simulink model "drone_obs"  (R2022a)
settings: Solver=VariableStepAuto  StartTime=0.0  StopTime=20  RelTol=1e-3
undefined symbols (not defined in the file): a1, a2, a3
settings Model: Creator=dfcpstage6  LastModifiedBy=dfcpstage6
settings DebuggingCC: UnconnectedInputMsg=warning  UnconnectedOutputMsg=warning  UnconnectedLineMsg=warning
settings RTWCC: DLArmComputeVersion=19.05

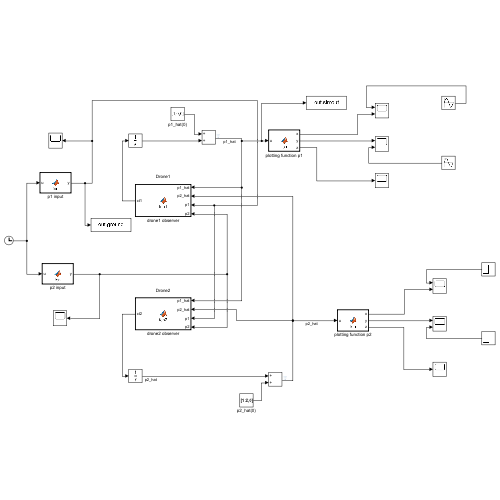
[thumbnail: Simulink's stored preview of the top-level diagram]
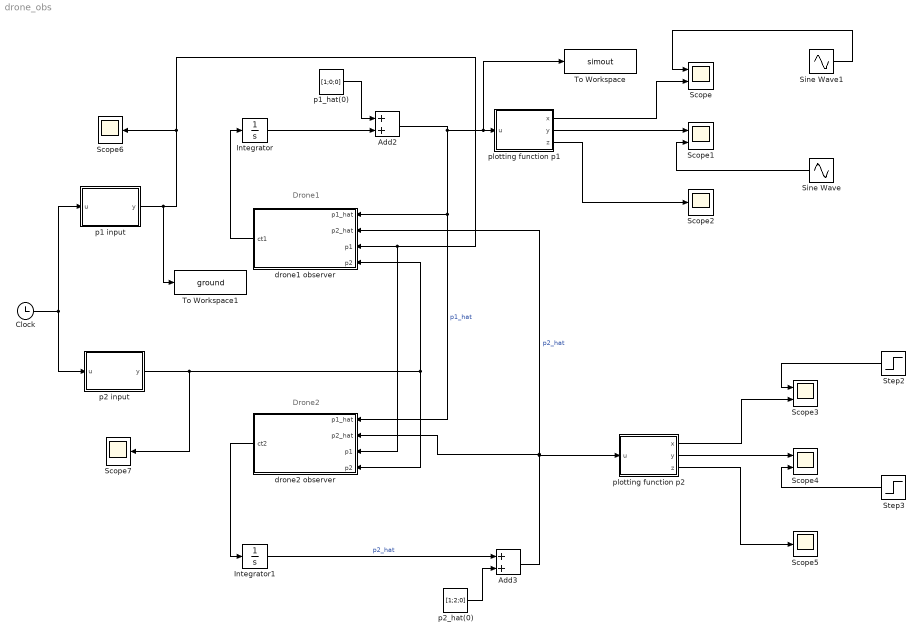
== system drone_obs ==
  note: Drone2
  note: Drone1
  Add2 : Sum
  Add3 : Sum
  Clock : Clock
  Integrator : Integrator
  Integrator1 : Integrator
  Scope{,1,3..4} (4 alike) : Scope  NumInputPorts=2
  Scope{2,5..7} (4 alike) : Scope
  Sine Wave : Sin  SampleTime=0
  Sine Wave1 : Sin  Phase=1.57  SampleTime=0
  Step2 : Step  Time=0.1  After=2  SampleTime=0
  Step3 : Step  Time=0.1  After=2  SampleTime=0
  To Workspace : ToWorkspace  VariableName=simout  SampleTime=-1
  To Workspace1 : ToWorkspace  VariableName=ground  SampleTime=-1
  drone1 observer : MATLAB Function  TreatAsAtomicUnit=on
  drone2 observer : MATLAB Function  TreatAsAtomicUnit=on
  p1 input : MATLAB Function  TreatAsAtomicUnit=on  SystemSampleTime=0.1
  p1_hat(0) : Constant  Value=[1;0;0]  VectorParams1D=off
  p2 input : MATLAB Function  TreatAsAtomicUnit=on  SystemSampleTime=0.1
  p2_hat(0) : Constant  Value=[1;2;0]  VectorParams1D=off
  plotting function p1 : MATLAB Function  TreatAsAtomicUnit=on
  plotting function p2 : MATLAB Function  TreatAsAtomicUnit=on
  wires:
  drone1 observer/1(ct1) -> Integrator/1
  drone2 observer/1(ct2) -> Integrator1/1
  Integrator/1 -> Add2/2
  Add2/1 -> drone2 observer/1(p1_hat), drone1 observer/1(p1_hat), To Workspace/1, plotting function p1/1(u)  "p1_hat"
  Integrator1/1 -> Add3/1  "p2_hat"
  p2_hat(0)/1 -> Add3/2
  p1_hat(0)/1 -> Add2/1
  plotting function p1/2(y) -> Scope1/1
  plotting function p1/3(z) -> Scope2/1
  plotting function p1/1(x) -> Scope/2
  p2 input/1(y) -> Scope7/1, drone1 observer/4(p2), drone2 observer/4(p2)
  p1 input/1(y) -> To Workspace1/1, drone2 observer/3(p1), drone1 observer/3(p1), Scope6/1
  plotting function p2/2(y) -> Scope4/1
  plotting function p2/3(z) -> Scope5/1
  Step2/1 -> Scope3/1
  Step3/1 -> Scope4/2
  plotting function p2/1(x) -> Scope3/2
  Add3/1 -> drone1 observer/2(p2_hat), drone2 observer/2(p2_hat), plotting function p2/1(u)  "p2_hat"
  Clock/1 -> p2 input/1(u), p1 input/1(u)
  Sine Wave1/1 -> Scope/1
  Sine Wave/1 -> Scope1/2

== matlab function drone_obs/drone2 observer ==
  data: p1_hat input; p2_hat input; ct2 output; a2 parameter; a3 parameter; p1 input; p2 input; a1 parameter
function ct2 = fcn2(p1_hat, p2_hat,a2, a3, p1, p2, a1)

% vel2 considering the second drone is just hovering in 2d space
    vel2 = [0;0;0];
%     vel2 = [2-p2(2); p2(1)-2 ;0];
    
%calculating the ranges manually
    d11 = norm(p1-a1);
    d13 = norm(p1-a3);
    d22 = norm(p2-a2);
    d23 = norm(p2-a3);
    q12 = norm(p1-p2);
    q21 = norm(p1-p2);
    
% our measured values
    y12 = d22^2 - d23^2 + norm(a3)^2 - norm(a2)^2;
    y22 = d23^2 + d13^2 - q21^2 - 2*norm(a3)^2;
    c23 = a3 - a2;
    
% controller gains
    k12 = c23;
    k22 = p1_hat - a3;
    
% correction terms
    ct2_1 = k12*(y12 - 2*(c23.')*p2_hat); 
    ct2_2 = k22*(y22 + 2*(a3.')*(p1_hat + p2_hat) - 2*(p1_hat.')*(p2_hat));
ct2 = vel2 + 1*ct2_1 + 1*ct2_2;

== matlab function drone_obs/drone1 observer ==
  data: p1_hat input; p2_hat input; ct1 output; p1 input; p2 input; a1 parameter; a2 parameter; a3 parameter
% function ct1 = fcn1(p1_hat, p2_hat ,a1, a3, d11, d13, d23, q21)
% 
% %     a1(1)
%     vel1 = [0;0;0];
%     y11 = d11^2 - d13^2 + norm(a3)^2 - norm(a1)^2;
%     y21 = d23^2 + d13^2 - q21^2 - 2*norm(a3)^2;
%     c13 = a3 - a1;
%     k11 = c13; k21 = p2_hat - a3;
%     ct1_1 = k11*(y11 - 2*(c13.')*p1_hat);
%     ct1_2 = k21*(y21 + 2*(a3.')*(p1_hat + p2_hat) - 2*(p1_hat.')*(p2_hat));
%         
%     N = ndims(ct1_1)
% ct1 = vel1 + ct1_1 + ct1_2;

function ct1 = fcn1(p1_hat, p2_hat ,p1, p2, a1, a2, a3)

% v1 for the drone if just hovering
%     vel1 = [0;0;0];

% v1 for the circular trajectory
    vel1 = [ -p1(2);p1(1); p1(3) ];
    
%calculating the ranges manually for now
    d11 = norm(p1-a1);
    d13 = norm(p1-a3);
    d22 = norm(p2-a2);
    d23 = norm(p2-a3);
    q12 = norm(p1-p2);
    q21 = norm(p1-p2);
    
% our measured values
    y11 = d11^2 - d13^2 + norm(a3)^2 - norm(a1)^2;
    y21 = d23^2 + d13^2 - q21^2 - 2*norm(a3)^2;
    
    c13 = a3 - a1;
% controller gains
    k11 = c13; k21 = p2_hat - a3;

% the correction terms finally added to ct1
    ct1_1 = k11*(y11 - 2*(c13.')*p1_hat);
    ct1_2 = k21*(y21 + 2*(a3.')*(p1_hat + p2_hat) - 2*(p1_hat.')*(p2_hat));
        
%     N = ndims(ct1_1)
ct1 = vel1 + 1*ct1_1 + 1*ct1_2;

== matlab function drone_obs/plotting function p1 ==
  data: u input; x output; y output; z output
function [x,y,z]= fcn(u)
%     x = u(1);
    x = u(1);
    y = u(2);
    z = u(3);
%     plot(x,y)
%     hold on
% y = u;

== matlab function drone_obs/plotting function p2 ==
  data: u input; x output; y output; z output
function [x,y,z]= fcn(u)
    x = u(1);
    y = u(2);
    z = u(3);
% y = u;

== matlab function drone_obs/p1 input ==
  data: y output; u input
function y = fcn(u)
%     t = linspace(0,100);
    xc = cos(1*u);
    yc = sin(1*u);
y = [xc;yc;0]; %generating p1 input for a circle trajectory

== matlab function drone_obs/p2 input ==
  data: y output; u input
function y = fcn(u)
%     t = linspace(0,5);
    xc = cos(u);
    yc = sin(u);
% y = xc;
y = [2;2;0]; % constant hover trajectory for p2
